simulink model "func5_c"  (R2019b)
settings: Solver=VariableStepAuto  StartTime=0.0  StopTime=10.0  RelTol=1e-3  EnableMultiTasking=on
libraries: templatized_input_5_lib x1
settings Model: Creator=abehbood  LastModifiedBy=abehbood
settings DataIOCC: ReturnWorkspaceOutputs=off
settings OptimizationCC: LifeSpan=inf
settings DebuggingCC: SFUnexpectedBacktrackingDiag=warning  SFNoUnconditionalDefaultTransitionDiag=warning  ArithmeticOperatorsInVariantConditions=warning
settings SFSimCC: SimUseLocalCustomCode=off  CustomCodeUndefinedFunction=UseInterfaceOnly
settings RTWCC: RTWUseLocalCustomCode=off
settings CodeAppCC: StateflowObjectComments=on
settings GRTTargetCC: TargetLangStandard=C89/C90 (ANSI)
settings ConfigComp: CovMetricSettings=dw  CovHtmlReporting=on  CovSaveCumulativeToWorkspaceVar=on  CovSaveSingleToWorkspaceVar=on  CovExternalEMLEnable=off

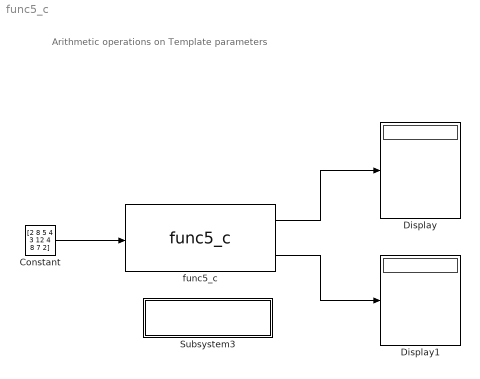
== system func5_c ==
  note: Arithmetic operations on
      | Template parameters
  Constant : Constant  Value=[2 8 5 4 3 12 4 8 7 2]  OutDataTypeStr=int16  SampleTime=1
  Display : Display
  Display1 : Display
  Subsystem3 : Subsystem
      settings: OpenFcn=xmcOpenFileEx
      mask Display: disp(sprintf('Double Click to open\nthe main header file'))
  func5_c : templatized_input_5_lib/func5_c  LibraryFunction=func5_c  IncludeFiles={'func5_c.h'}  SourceFiles={}  IncludeDirectories={}  TemplateParams={'int NUMOFELEMENTS'}  FunctionParamTypes={xmcDataType('void'); xmcDataType('int16_t'); xmcDataType('int16_t'); xmcDataType('int16_t')}  FunctionParamPassbys={0.000000000000000000e+00; 0.000000000000000000e+00; 0.000000000000000000e+00; 0.000000000000000000e+00}  FunctionParamDimensions={'1'; '[NUMOFELEMENTS]'; '[NUMOFELEMENTS / 2]'; '[2 * NUMOFELEMENTS - 15]'}  FunctionParamNames={'return'; 'in'; 'out0'; 'out1'}  FunctionParamDir={0.000000000000000000e+00; 1.000000000000000000e+00; 2.000000000000000000e+00; 2.000000000000000000e+00}  FunctionParamSupportsStreaming={false; false; false; false}  BufferDepth={'0'}  FunctionParamValues={'0'; '0'; '0'; '0'}  ThroughputFactors={''}
  wires:
  func5_c/2 -> Display1/1
  func5_c/1 -> Display/1
  Constant/1 -> func5_c/1

== system func5_c/Subsystem3 ==
